simulink model "xiankong05_nolinear"  (Simulink 9.0)
settings: Solver=VariableStepAuto  StartTime=0.0  StopTime=10.0  RelTol=1e-3
values from neighbouring files (symbols this model uses):
  G2_s = sym2poly(d)    [xiankong05.m]
  G2_z = sym2poly(n)    [xiankong05.m]
  G3_s = sym2poly(d)    [xiankong05.m]
  G3_z = sym2poly(n)    [xiankong05.m]
  K2 = K(3)    [xiankong03.m]    (also in xiankong03v2.m; xiankong03v4.m; xiankong04.m; xiankong04v2.m)
  s_max = s_value    (= 10)    [xiankong01.m]    (also in xiankong02.m; xiankong03.m; xiankong03v2.m; xiankong03v4.m = 0.01)
  s_min = -s_value    (= -10)    [xiankong01.m]    (also in xiankong02.m; xiankong03.m; xiankong03v2.m; xiankong03v4.m = -0.01)
  u_k = 10    [xiankong01.m]    (also in xiankong02.m; xiankong05.m = 1)
undefined symbols (not defined in the file or in its folder): G0_s, G0_z
settings Model: Creator=wulin  LastModifiedBy=wulin
settings DataIOCC: SaveFormat=Dataset
settings OptimizationCC: LifeSpan=auto
settings DebuggingCC: UnderspecifiedInitializationDetection=Simplified  MergeDetectMultiDrivingBlocksExec=error  SFUnexpectedBacktrackingDiag=error  SFNoUnconditionalDefaultTransitionDiag=error  SFExecutionAtInitializationDiag=warning
settings HardwareCC: ProdBitPerPointer=64  ProdBitPerSizeT=64  ProdBitPerPtrDiffT=64  ProdLargestAtomicFloat=Float  ProdIntDivRoundTo=Zero  ProdEndianess=LittleEndian  ProdWordSize=64  ProdHWDeviceType=Intel->x86-64 (Windows64)
settings ModelReferenceCC: PropagateSignalLabelsOutOfModel=on
settings CodeAppCC: StateflowObjectComments=off
settings GRTTargetCC: TargetLangStandard=C99 (ISO)
settings ConfigComp: CovMetricSettings=dwe  CovHtmlReporting=off  CovSaveCumulativeToWorkspaceVar=off  CovSaveSingleToWorkspaceVar=off  CovExternalEMLEnable=on

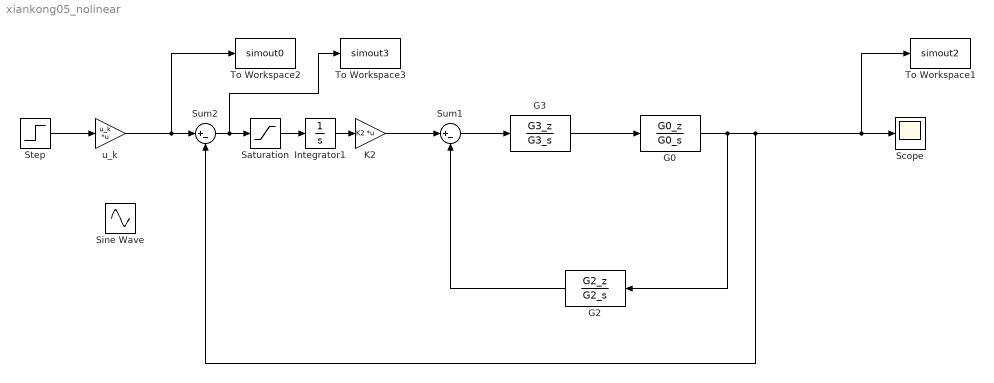
== system xiankong05_nolinear ==
  G0 : TransferFcn  Numerator=G0_z  Denominator=G0_s
  G2 : TransferFcn  Numerator=G2_z  Denominator=G2_s
  G3 : TransferFcn  Numerator=G3_z  Denominator=G3_s
  Integrator1 : Integrator
  K2 : Gain  Gain=K2  Multiplication=Matrix(K*u) (u vector)
  Saturation : Saturate  UpperLimit=s_max  LowerLimit=s_min
  Scope : Scope
  Sine Wave : Sin  SampleTime=0
  Step : Step  SampleTime=0
  Sum1 : Sum  Inputs=|+-
  Sum2 : Sum  Inputs=|+-
  To Workspace1 : ToWorkspace  VariableName=simout2  SampleTime=-1
  To Workspace2 : ToWorkspace  VariableName=simout0  SampleTime=-1
  To Workspace3 : ToWorkspace  VariableName=simout3  SampleTime=-1
  u_k : Gain  Gain=u_k  Multiplication=Matrix(K*u) (u vector)
  wires:
  Integrator1/1 -> K2/1
  K2/1 -> Sum1/1
  G0/1 -> To Workspace1/1, Scope/1, Sum2/2, G2/1
  G2/1 -> Sum1/2
  G3/1 -> G0/1
  Sum1/1 -> G3/1
  u_k/1 -> Sum2/1, To Workspace2/1
  Sum2/1 -> To Workspace3/1, Saturation/1
  Saturation/1 -> Integrator1/1
  Step/1 -> u_k/1
